simulink model "WingLoop_Controller"  (R2025a)
settings: Solver=ode4  StartTime=0.0  StopTime=T_sim  FixedStep=0.1  RelTol=1e-3
InitFcn:
  | WL_init_callback
values from neighbouring files (symbols this model uses):
  Dt_asw = 0.1    [WingLoop_Simulink_Testrun.m]
  u_trim = [0, F2ref, F3ref, 0, E2ref, E2ref]    [WingLoop_Simulink_Testrun.m]
settings Model: SimulationMode=accelerator  Creator=lpmat  LastModifiedBy=lpmat

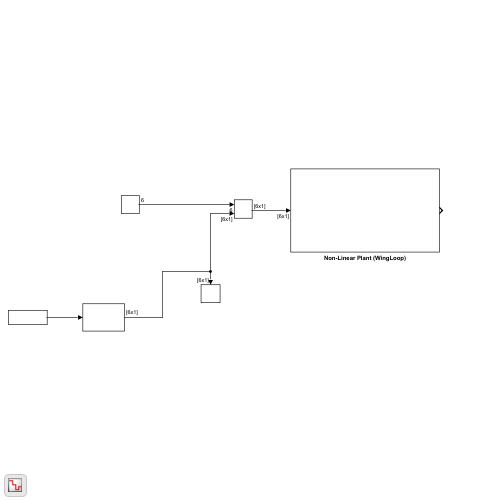
[thumbnail: Simulink's stored preview of the top-level diagram]
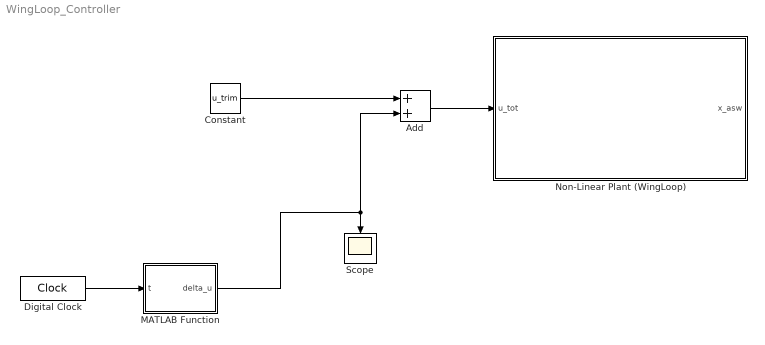
== system WingLoop_Controller ==
  Add : Sum
  Constant : Constant  Value=u_trim
  Digital Clock : DigitalClock  SampleTime=Dt_asw
  MATLAB Function : MATLAB Function  TreatAsAtomicUnit=on
  Non-Linear Plant (WingLoop) : Subsystem
      mask Display: image('Screenshot 2026-03-18 123158.png');
  Scope : Scope
      settings: ActiveDisplayYMinimum=-1  ActiveDisplayYMaximum=1
  wires:
  Constant/1 -> Add/1
  Add/1 -> Non-Linear Plant (WingLoop)/1(u_tot)
  Digital Clock/1 -> MATLAB Function/1(t)
  MATLAB Function/1(delta_u) -> Add/2, Scope/1

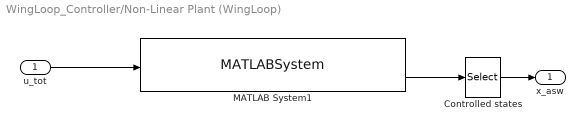
== system WingLoop_Controller/Non-Linear Plant (WingLoop) ==
  u_tot : Inport
  Controlled states : Selector  InputPortWidth=1888  IndexOptions=Index vector (dialog)  Indices=[1:1882]  OutputSizes=1
  MATLAB System1 : MATLABSystem  System=AswingPlant  ServerHost=localhost  ServerPort=5005  NumModalStates=91  NumPhysicalStates=1888  ConnectRetries=60  SocketTimeout=60  SimulateUsing=Interpreted execution
      mask Type: AswingPlant
  x_asw : Outport
  wires:
  MATLAB System1/2 -> Controlled states/1
  u_tot/1 -> MATLAB System1/1
  Controlled states/1 -> x_asw/1

== matlab function WingLoop_Controller/MATLAB Function ==
  data: t input; delta_u output
function delta_u = generate_validation_cmd(t)
    % Parametri della manovra
    t_start = 1.0;  % Inizio incremento a 1 secondo
    tau = 1.0;      % Costante di tempo (velocità della curva)
    
    % Inizializziamo il vettore delta_u (6 canali)
    delta_u = zeros(6, 1);
    
    if t >= t_start
        % Calcolo della dinamica esponenziale: 1 - exp(-t/tau)
        % Arriva al 99% del target in circa 5*tau secondi
        dinamica = (1.0 - exp(-(t - t_start) / tau));
        
        % Canale 2: Flap (+1 grado)
        delta_u(2) = 1.0 * dinamica;
        
        
    end
end
